simulink library "hdlsllibUNLOCKED"  (R2019a)
settings: Solver=ode45  StartTime=0.0  StopTime=10.0  RelTol=1e-3  EnableMultiTasking=on
values from neighbouring files (symbols this model uses):
  freerun = strcmp(get_param(blk, 'CountType'), 'Free running')    [hdlblkmask_counter.m]
  maxval_sc = countrange(2)    [hdlblkmask_counter.m]
  samptime = -1    [hdlblkmask_counter.m]
undefined symbols (not defined in the file or in its folder): a, b, c, Dialog, DiscIntNeverNeededParam, Floor, HDLStatusEnum, jsin, magnitude, message, Newton, NumBits1, NumBits2, Raphson, Slope1, Slope2
libraries: simulink x70, $bdroot x5, hdlmdlgenlib x1, hdlsllib_helper x1
(part 2 of 3)

== system hdlsllibUNLOCKED/Discrete/Unit Delay Enabled Resettable Synchronous ==
  u : Inport
  E : Inport  Port=2
  R : Inport  Port=3
  Unit Delay Enabled Resettable : Subsystem
  y : Outport
  wires:
  u/1 -> Unit Delay Enabled Resettable/1(u)
  E/1 -> Unit Delay Enabled Resettable/2(E)
  R/1 -> Unit Delay Enabled Resettable/3(R)
  Unit Delay Enabled Resettable/1(y) -> y/1

== system hdlsllibUNLOCKED/Discrete/Unit Delay Resettable Synchronous ==
  u : Inport
  R : Inport  Port=2
  Unit Delay Resettable : Subsystem
  y : Outport
  wires:
  u/1 -> Unit Delay Resettable/1(u)
  R/1 -> Unit Delay Resettable/2(R)
  Unit Delay Resettable/1(y) -> y/1

== system hdlsllibUNLOCKED/HDL Subsystems/Enabled Synchronous Subsystem ==
  In1 : Inport
  Enable : EnablePort
  State Control : StateControl  StateControl=Synchronous
  Out1 : Outport
  wires:
  In1/1 -> Out1/1

== system hdlsllibUNLOCKED/HDL Subsystems/Resettable Synchronous Subsystem ==
  In1 : Inport
  Reset : ResetPort  DisableCoverage=on  ResetTriggerType=level hold
  State Control : StateControl  StateControl=Synchronous
  Out1 : Outport
  wires:
  In1/1 -> Out1/1

== system hdlsllibUNLOCKED/HDL Subsystems/Synchronous Subsystem ==
  In1 : Inport
  State Control : StateControl  StateControl=Synchronous
  Out1 : Outport
  wires:
  In1/1 -> Out1/1

== system hdlsllibUNLOCKED/HDL Operations/Deserializer1D ==
  S : Inport
  Delay : Delay  DelayLength=1  InitialCondition=0
  EnumToIntConverter : MATLAB Function  TreatAsAtomicUnit=on
  HDL1DDs : MATLABSystem  System=hdl.deserializer1D  Ratio=Ratio  IdleCycles=IdleCycles  InitialCondition=0  StartInPortEnb=off  ValidInPortEnb=off  SimulateUsing=Code generation
      mask Type: hdl.deserializer1D
      mask Display:
      | disp(['Deserializer' char(10) '1D']);
      | port_label('input',1,'dataIn');
      | port_label('input',2,'startIn');
      | port_label('input',3,'validIn');
      | port_label('output',1,'dataOut');
      | port_label('output',2,'validOut');
  IntToEnumConverter : MATLAB Function  TreatAsAtomicUnit=on
  Terminator : Terminator
  const_startIn : Constant  OutDataTypeStr=boolean
  const_validIn : Constant  OutDataTypeStr=boolean
  rateTrans : RateTransition  OutPortSampleTimeOpt=Multiple of input port sample time  OutPortSampleTimeMultiple=1 + 0  OutPortSampleTime=1
  rateTrans1 : RateTransition  OutPortSampleTimeOpt=Multiple of input port sample time  OutPortSampleTimeMultiple=1 + 0  OutPortSampleTime=1
  P : Outport
  wires:
  Delay/1 -> IntToEnumConverter/1(dataIn)
  S/1 -> Delay/1, EnumToIntConverter/1(dataIn)
  rateTrans/1 -> P/1
  HDL1DDs/2 -> rateTrans1/1
  rateTrans1/1 -> Terminator/1
  EnumToIntConverter/1(deserializer_preProcessed) -> HDL1DDs/1
  HDL1DDs/1 -> IntToEnumConverter/2(dataOut)
  IntToEnumConverter/1(deserializer_PostProcessed) -> rateTrans/1
  const_startIn/1 -> HDL1DDs/2
  const_validIn/1 -> HDL1DDs/3

== system hdlsllibUNLOCKED/HDL Operations/Multiply-Accumulate ==
  a : Inport
  b : Inport  Port=2
  streamingMAC_with_counter : Subsystem  Commented=on  mask{initValueSetting=Dialog, initValue=initValue3, num_samples_internal=num_samples, typeinfo=Inherit: Inherit via back propagation, RndMeth=Floor}
      mask prompts: num_samples_internal "Number of Samples:"; typeinfo "Output data type:"; RndMeth "Integer rounding mode"
      mask init:
      | hdlblkmask_streaming_internal(gcb, initValueSetting, initValue, num_samples_internal)
      mask TypeOptions initValueSetting: Dialog | Input port
      mask Callback initValueSetting: hdlblkmask_streaming_internal_cb(gcb)
      mask TypeOptions RndMeth: Multiply-Add/RndMeth
      mask DialogControl Container3 Prompt: Data
      mask DialogControl Control2 Prompt: (Add text here)
      mask DialogControl Control3 Prompt: Source
      mask DialogControl Control4 Prompt: Value
      mask DialogControl Control5 Prompt: Bias:
  streamingMAC_without_counter : Subsystem  Commented=on  mask{initValueSetting=Dialog, initValue=initValue2, typeinfo=Inherit: Inherit via back propagation, RndMeth=Floor}
      mask prompts: typeinfo "Output data type:"; RndMeth "Integer rounding mode"
      mask init:
      | hdlblkmask_streaming_internal(gcb,initValueSetting,initValue)
      mask TypeOptions initValueSetting: Dialog | Input port
      mask Callback initValueSetting: hdlblkmask_streaming_internal_cb(gcb)
      mask TypeOptions RndMeth: Multiply-Add/RndMeth
      mask DialogControl Container3 Prompt: Data
      mask DialogControl Control2 Prompt: (Add text here)
      mask DialogControl Control3 Prompt: Source
      mask DialogControl Control4 Prompt: Value
      mask DialogControl Control5 Prompt: Bias:
  vectorMAC : Subsystem  mask{dim=-1, initValueSetting=Dialog, initValue=initValue, parallel=off, AccumDataTypeStr=Inherit: Inherit via internal rule, RndMeth=Floor, DoSatur=off}
      mask prompts: dim "Specify input dimensions"; parallel "Use fully parallel implementation"; AccumDataTypeStr "Simulink:blkprm_prompts:OUTPUT_UNIFIEDDATATYPE"; RndMeth "Simulink:blkprm_prompts:SPP_RndMeth_ID"; DoSatur "Simulink:blkprm_prompts:AllBlksSaturate"
      mask init:
      | hdlblkmask_mac(gcb, initValueSetting, initValue)
      mask TypeOptions initValueSetting: Dialog | Input port
      mask Callback initValueSetting: hdlblkmask_mac_cb(gcb);
      mask TypeOptions AccumDataTypeStr: Sum/AccumDataTypeStr
      mask TypeOptions RndMeth: Sum/RndMeth
      mask TypeOptions DoSatur: Sum/SaturateOnIntegerOverflow
      mask DialogControl Container3 Prompt: Data
      mask DialogControl Control3 Prompt: (Add text here)
      mask DialogControl Control4 Prompt: Source
      mask DialogControl Control5 Prompt: Value
      mask DialogControl Control2 Prompt: Bias:
      mask DialogControl AccumDataTypeStr Prompt: Output data type:
      mask DialogControl RndMeth Prompt: Integer rounding mode:
      mask DialogControl DoSatur Prompt: Saturate on integer overflow
      mask Display:
      | maskVal = get_param(gcb,'MaskValues');
      | initValueSetting = maskVal{2};
      | if(strcmp(initValueSetting,'Input port'))
      |     port_label('input', 1, 'a');
      |     port_label('input', 2, 'b');
      |     port_label('input', 3, 'c');
      |     disp([char(8721),'a(i)*b(i)+c'])
      | elseif(initValue ~= 0)
      |     port_label('input', 1, 'a');
      |     port_label('input', 2, 'b');
      |     disp([char(8721),'a(i)*b(i)+k'])
      | else
      |     port_label('input', 1, 'a');
      |     port_label('input', 2, 'b');
      |     disp([char(8721),'a(i)*b(i)'])
      | end
  dataOut : Outport
  wires:
  a/1 -> vectorMAC/1(In1)
  b/1 -> vectorMAC/2(In2)
  vectorMAC/1(Out1) -> dataOut/1

== system hdlsllibUNLOCKED/HDL Operations/Multiply-Add ==
  a : Inport
  b : Inport  Port=2
  c : Inport  Port=3
  Product : Product
  Sum : Sum  OutDataTypeStr=datatype
  Out : Outport
  wires:
  c/1 -> Sum/1
  a/1 -> Product/1
  b/1 -> Product/2
  Sum/1 -> Out/1
  Product/1 -> Sum/2

== system hdlsllibUNLOCKED/HDL Operations/Serializer1D ==
  P : Inport
  EnumToIntConverter : MATLAB Function  TreatAsAtomicUnit=on
  HDL1DSe : MATLABSystem  System=hdl.serializer1D  Ratio=Ratio  IdleCycles=IdleCycles  SimulateUsing=Code generation
      mask Type: hdl.serializer1D
      mask Display:
      | disp(['Serializer' char(10) '1D']);
      | port_label('input',1,'dataIn');
      | port_label('input',2,'validIn');
      | port_label('output',1,'dataOut');
      | port_label('output',2,'startOut');
      | port_label('output',3,'validOut');
  IntToEnumConverter : MATLAB Function  TreatAsAtomicUnit=on
  Terminator : Terminator
  Terminator1 : Terminator
  const_validIn : Constant  OutDataTypeStr=boolean
  rateTrans : RateTransition  Integrity=off  OutPortSampleTimeOpt=Multiple of input port sample time  OutPortSampleTimeMultiple=1/(1 + 0)  OutPortSampleTime=1
  rateTrans1 : RateTransition  Integrity=off  OutPortSampleTimeOpt=Multiple of input port sample time  OutPortSampleTimeMultiple=1/(1 + 0)  OutPortSampleTime=1
  S : Outport
  wires:
  P/1 -> rateTrans/1
  rateTrans/1 -> IntToEnumConverter/1(dataIn), EnumToIntConverter/1(dataIn)
  HDL1DSe/2 -> Terminator/1
  HDL1DSe/3 -> Terminator1/1
  rateTrans1/1 -> HDL1DSe/2
  const_validIn/1 -> rateTrans1/1
  EnumToIntConverter/1(serializer_preProcessed) -> HDL1DSe/1
  HDL1DSe/1 -> IntToEnumConverter/2(dataOut)
  IntToEnumConverter/1(serializer_PostProcessed) -> S/1

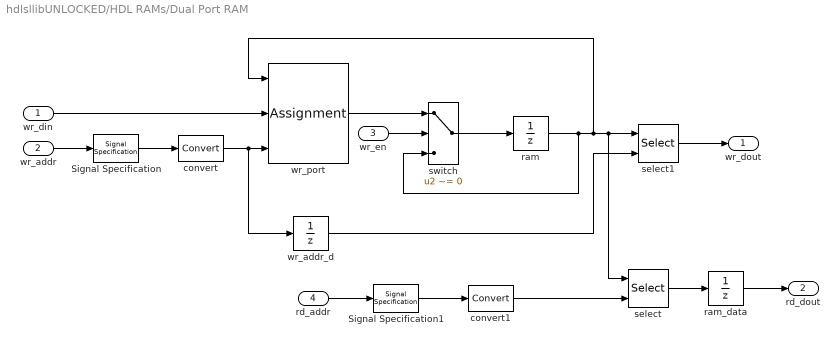
== system hdlsllibUNLOCKED/HDL RAMs/Dual Port RAM ==
  wr_din : Inport
  wr_addr : Inport  Port=2
  wr_en : Inport  Port=3  OutDataTypeStr=boolean
  rd_addr : Inport  Port=4
  Signal Specification : SignalSpecification  OutDataTypeStr=fixdt(0,ram_size,0)  Dimensions=1
  Signal Specification1 : SignalSpecification  OutDataTypeStr=fixdt(0,ram_size,0)  Dimensions=1
  convert : DataTypeConversion
  convert1 : DataTypeConversion
  ram : UnitDelay  SampleTime=-1  HasFrameUpgradeWarning=on
  ram_data : UnitDelay  SampleTime=-1  HasFrameUpgradeWarning=on
  select : Selector  IndexMode=Zero-based  InputPortWidth=2^ram_size  IndexOptions=Index vector (port)  Indices=[1 3]  OutputSizes=1
  select1 : Selector  IndexMode=Zero-based  InputPortWidth=2^ram_size  IndexOptions=Index vector (port)  Indices=[1 3]  OutputSizes=1
  switch : Switch  Criteria=u2 ~= 0
  wr_addr_d : UnitDelay  SampleTime=-1  HasFrameUpgradeWarning=on
  wr_port : Assignment  IndexMode=Zero-based  IndexOptions=Index vector (port)  Indices=1  OutputSizes=[1 1]
  wr_dout : Outport
  rd_dout : Outport  Port=2
  wires:
  Signal Specification1/1 -> convert1/1
  wr_addr_d/1 -> select1/2
  select1/1 -> wr_dout/1
  convert1/1 -> select/2
  convert/1 -> wr_addr_d/1, wr_port/3
  select/1 -> ram_data/1
  rd_addr/1 -> Signal Specification1/1
  wr_en/1 -> switch/2
  wr_din/1 -> wr_port/2
  ram/1 -> switch/3, select1/1, select/1, wr_port/1
  switch/1 -> ram/1
  wr_port/1 -> switch/1
  wr_addr/1 -> Signal Specification/1
  Signal Specification/1 -> convert/1
  ram_data/1 -> rd_dout/1

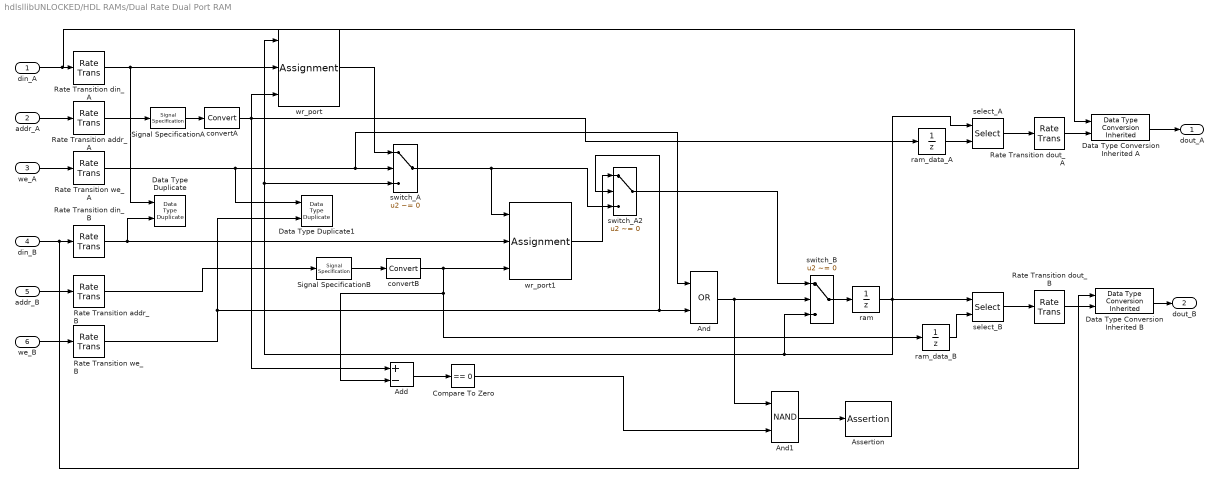
== system hdlsllibUNLOCKED/HDL RAMs/Dual Rate Dual Port RAM ==
  din_A : Inport
  addr_A : Inport  Port=2
  we_A : Inport  Port=3  OutDataTypeStr=boolean
  din_B : Inport  Port=4
  addr_B : Inport  Port=5
  we_B : Inport  Port=6  OutDataTypeStr=boolean
  Add : Sum  Inputs=+-
  And : Logic  Operator=OR  AllPortsSameDT=off  OutDataTypeStr=boolean
  And1 : Logic  Operator=NAND  AllPortsSameDT=off  OutDataTypeStr=boolean
  Assertion : Assertion
  Compare To Zero : simulink/Logic and Bit Operations/Compare To Zero  relop===  OutDataTypeStr=boolean
  Data Type Conversion Inherited A : simulink/Signal Attributes/Data Type Conversion Inherited  ConvertRealWorld=Real World Value  DoSatur=off
      settings: SourceProductName=Simulink  SourceProductBaseCode=SL
  Data Type Conversion Inherited B : simulink/Signal Attributes/Data Type Conversion Inherited  ConvertRealWorld=Real World Value  DoSatur=off
      settings: SourceProductName=Simulink  SourceProductBaseCode=SL
  Data Type Duplicate : DataTypeDuplicate
  Data Type Duplicate1 : DataTypeDuplicate
  Rate Transition addr_A : RateTransition  Integrity=off
  Rate Transition addr_B : RateTransition  Integrity=off
  Rate Transition din_A : RateTransition  Integrity=off
  Rate Transition din_B : RateTransition  Integrity=off
  Rate Transition dout_A : RateTransition  Integrity=off
  Rate Transition dout_B : RateTransition  Integrity=off
  Rate Transition we_A : RateTransition  Integrity=off
  Rate Transition we_B : RateTransition  Integrity=off
  Signal SpecificationA : SignalSpecification  OutDataTypeStr=fixdt(0,ram_size,0)  Dimensions=1
  Signal SpecificationB : SignalSpecification  OutDataTypeStr=fixdt(0,ram_size,0)  Dimensions=1
  convertA : DataTypeConversion
  convertB : DataTypeConversion
  ram : UnitDelay  SampleTime=-1  HasFrameUpgradeWarning=on
  ram_data_A : UnitDelay  SampleTime=-1  HasFrameUpgradeWarning=on
  ram_data_B : UnitDelay  SampleTime=-1  HasFrameUpgradeWarning=on
  select_A : Selector  IndexMode=Zero-based  InputPortWidth=2^ram_size  IndexOptions=Index vector (port)  Indices=[1 3]  OutputSizes=1
  select_B : Selector  IndexMode=Zero-based  InputPortWidth=2^ram_size  IndexOptions=Index vector (port)  Indices=[1 3]  OutputSizes=1
  switch_A : Switch  Criteria=u2 ~= 0
  switch_A2 : Switch  Criteria=u2 ~= 0
  switch_B : Switch  Criteria=u2 ~= 0
  wr_port : Assignment  IndexMode=Zero-based  IndexOptions=Index vector (port)  Indices=1  OutputSizes=[1 1]
  wr_port1 : Assignment  IndexMode=Zero-based  IndexOptions=Index vector (port)  Indices=1  OutputSizes=[1 1]
  dout_A : Outport
  dout_B : Outport  Port=2
  wires:
  we_A/1 -> Rate Transition we_A/1
  select_A/1 -> Rate Transition dout_A/1
  switch_A2/1 -> switch_B/1
  And1/1 -> Assertion/1
  Signal SpecificationA/1 -> convertA/1
  Signal SpecificationB/1 -> convertB/1
  din_B/1 -> Data Type Conversion Inherited B/1, Rate Transition din_B/1
  switch_B/1 -> ram/1
  addr_B/1 -> Rate Transition addr_B/1
  convertA/1 -> ram_data_A/1, wr_port/3, Add/1
  we_B/1 -> Rate Transition we_B/1
  ram/1 -> select_B/1, switch_B/3, switch_A/3, wr_port/1, select_A/1
  wr_port/1 -> switch_A/1
  And/1 -> And1/1, switch_B/2
  wr_port1/1 -> switch_A2/1
  Add/1 -> Compare To Zero/1
  Compare To Zero/1 -> And1/2
  Rate Transition we_B/1 -> switch_A2/2, And/2, Data Type Duplicate1/2
  switch_A/1 -> wr_port1/1, switch_A2/3
  Rate Transition addr_B/1 -> Signal SpecificationB/1
  select_B/1 -> Rate Transition dout_B/1
  ram_data_B/1 -> select_B/2
  Rate Transition we_A/1 -> Data Type Duplicate1/1, And/1, switch_A/2
  ram_data_A/1 -> select_A/2
  Rate Transition din_A/1 -> Data Type Duplicate/1, wr_port/2
  convertB/1 -> ram_data_B/1, Add/2, wr_port1/3
  din_A/1 -> Data Type Conversion Inherited A/1, Rate Transition din_A/1
  Rate Transition din_B/1 -> wr_port1/2, Data Type Duplicate/2
  addr_A/1 -> Rate Transition addr_A/1
  Rate Transition addr_A/1 -> Signal SpecificationA/1
  Rate Transition dout_B/1 -> Data Type Conversion Inherited B/2
  Data Type Conversion Inherited B/1 -> dout_B/1
  Rate Transition dout_A/1 -> Data Type Conversion Inherited A/2
  Data Type Conversion Inherited A/1 -> dout_A/1

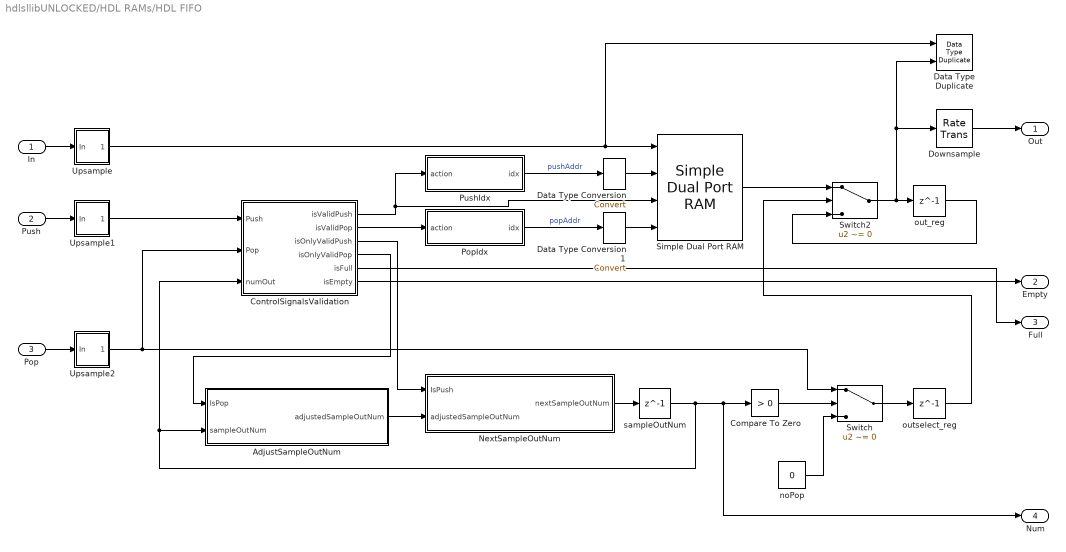
== system hdlsllibUNLOCKED/HDL RAMs/HDL FIFO ==
  In : Inport  PortDimensions=1
  Push : Inport  Port=2  PortDimensions=1
  Pop : Inport  Port=3  PortDimensions=1
  AdjustSampleOutNum : Subsystem
  Compare To Zero : simulink/Logic and Bit Operations/Compare To Zero  relop=>  OutDataTypeStr=boolean
  ControlSignalsValidation : Subsystem
  Data Type Duplicate : DataTypeDuplicate
  Data Type Conversion : DataTypeConversion
  Data Type Conversion1 : DataTypeConversion
  Downsample : RateTransition  OutPortSampleTimeOpt=Multiple of input port sample time  OutPortSampleTimeMultiple=ratio
  NextSampleOutNum : Subsystem
  PopIdx : Subsystem
  PushIdx : Subsystem
  Simple Dual Port RAM : $bdroot/HDL RAMs/Simple Dual Port RAM  ram_size=4
  Switch : Switch  Criteria=u2 ~= 0
  Switch2 : Switch  Criteria=u2 ~= 0
  Upsample : Subsystem
  Upsample1 : Subsystem
  Upsample2 : Subsystem
  noPop : Constant  Value=0
  out_reg : Delay  DelayLength=1  InitialCondition=0
  outselect_reg : Delay  DelayLength=1  InitialCondition=0
  sampleOutNum : Delay  DelayLength=1  InitialCondition=0
  Out : Outport  PortDimensions=1
  Empty : Outport  Port=2  PortDimensions=1
  Full : Outport  Port=3  PortDimensions=1
  Num : Outport  Port=4  PortDimensions=1
  wires:
  Downsample/1 -> Out/1
  Upsample2/1(Out) -> ControlSignalsValidation/2(Pop), Switch/1
  Upsample1/1(Out) -> ControlSignalsValidation/1(Push)
  Upsample/1(Out) -> Data Type Duplicate/1, Simple Dual Port RAM/1
  Simple Dual Port RAM/1 -> Switch2/1
  sampleOutNum/1 -> ControlSignalsValidation/3(numOut), AdjustSampleOutNum/2(sampleOutNum), Num/1, Compare To Zero/1
  AdjustSampleOutNum/1(adjustedSampleOutNum) -> NextSampleOutNum/2(adjustedSampleOutNum)
  NextSampleOutNum/1(nextSampleOutNum) -> sampleOutNum/1
  ControlSignalsValidation/2(isValidPop) -> PopIdx/1(action)
  out_reg/1 -> Switch2/3
  In/1 -> Upsample/1(In)
  outselect_reg/1 -> Switch2/2
  Switch/1 -> outselect_reg/1
  PushIdx/1(idx) -> Data Type Conversion/1  "pushAddr"
  PopIdx/1(idx) -> Data Type Conversion1/1  "popAddr"
  Switch2/1 -> Data Type Duplicate/2, Downsample/1, out_reg/1
  Compare To Zero/1 -> Switch/2
  noPop/1 -> Switch/3
  ControlSignalsValidation/4(isOnlyValidPop) -> AdjustSampleOutNum/1(IsPop)
  ControlSignalsValidation/5(isFull) -> Full/1
  ControlSignalsValidation/3(isOnlyValidPush) -> NextSampleOutNum/1(IsPush)
  ControlSignalsValidation/6(isEmpty) -> Empty/1
  Data Type Conversion1/1 -> Simple Dual Port RAM/4
  Data Type Conversion/1 -> Simple Dual Port RAM/2
  ControlSignalsValidation/1(isValidPush) -> PushIdx/1(action), Simple Dual Port RAM/3
  Push/1 -> Upsample1/1(In)
  Pop/1 -> Upsample2/1(In)

== system hdlsllibUNLOCKED/HDL RAMs/Simple Dual Port RAM ==
  wr_din : Inport
  wr_addr : Inport  Port=2
  wr_en : Inport  Port=3  OutDataTypeStr=boolean
  rd_addr : Inport  Port=4
  Signal Specification : SignalSpecification  OutDataTypeStr=fixdt(0,ram_size,0)  Dimensions=1
  Signal Specification1 : SignalSpecification  OutDataTypeStr=fixdt(0,ram_size,0)  Dimensions=1
  convert : DataTypeConversion
  convert1 : DataTypeConversion
  ram : UnitDelay  SampleTime=-1  HasFrameUpgradeWarning=on
  ram_data : UnitDelay  SampleTime=-1  HasFrameUpgradeWarning=on
  select : Selector  IndexMode=Zero-based  InputPortWidth=2^ram_size  IndexOptions=Index vector (port)  Indices=[1 3]  OutputSizes=1
  switch : Switch  Criteria=u2 ~= 0
  wr_port : Assignment  IndexMode=Zero-based  IndexOptions=Index vector (port)  Indices=1  OutputSizes=[1 1]
  rd_dout : Outport
  wires:
  wr_port/1 -> switch/1
  switch/1 -> ram/1
  ram/1 -> wr_port/1, select/1, switch/3
  wr_din/1 -> wr_port/2
  wr_en/1 -> switch/2
  wr_addr/1 -> Signal Specification/1
  rd_addr/1 -> Signal Specification1/1
  select/1 -> ram_data/1
  convert/1 -> wr_port/3
  convert1/1 -> select/2
  Signal Specification/1 -> convert/1
  Signal Specification1/1 -> convert1/1
  ram_data/1 -> rd_dout/1

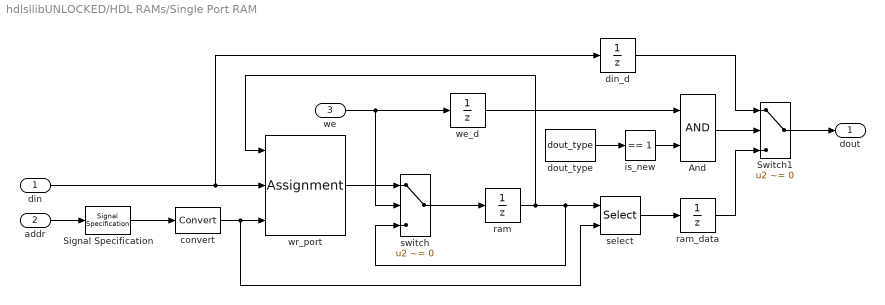
== system hdlsllibUNLOCKED/HDL RAMs/Single Port RAM ==
  din : Inport
  addr : Inport  Port=2
  we : Inport  Port=3  OutDataTypeStr=boolean
  And : Logic  AllPortsSameDT=off  OutDataTypeStr=boolean
  Signal Specification : SignalSpecification  OutDataTypeStr=fixdt(0,ram_size,0)  Dimensions=1
  Switch1 : Switch  Criteria=u2 ~= 0
  convert : DataTypeConversion
  din_d : UnitDelay  SampleTime=-1  HasFrameUpgradeWarning=on
  dout_type : Constant  Value=dout_type
  is_new : simulink/Logic and Bit Operations/Compare To Constant  relop===  const=1  OutDataTypeStr=boolean  ZeroCross=off
  ram : UnitDelay  SampleTime=-1  HasFrameUpgradeWarning=on
  ram_data : UnitDelay  SampleTime=-1  HasFrameUpgradeWarning=on
  select : Selector  IndexMode=Zero-based  InputPortWidth=2^ram_size  IndexOptions=Index vector (port)  Indices=[1 3]  OutputSizes=1
  switch : Switch  Criteria=u2 ~= 0
  we_d : UnitDelay  SampleTime=-1  HasFrameUpgradeWarning=on
  wr_port : Assignment  IndexMode=Zero-based  IndexOptions=Index vector (port)  Indices=1  OutputSizes=[1 1]
  dout : Outport
  wires:
  wr_port/1 -> switch/1
  switch/1 -> ram/1
  ram/1 -> switch/3, wr_port/1, select/1
  din/1 -> wr_port/2, din_d/1
  we/1 -> switch/2, we_d/1
  addr/1 -> Signal Specification/1
  select/1 -> ram_data/1
  convert/1 -> wr_port/3, select/2
  Signal Specification/1 -> convert/1
  Switch1/1 -> dout/1
  din_d/1 -> Switch1/1
  And/1 -> Switch1/2
  ram_data/1 -> Switch1/3
  dout_type/1 -> is_new/1
  is_new/1 -> And/2
  we_d/1 -> And/1

== system hdlsllibUNLOCKED/Logic and Bit Operations/Bit Concat ==
  u1 : Inport
  u2 : Inport  Port=2
  Bit Concat2 : hdlmdlgenlib/Bit Concat2
      settings: SourceProductName=Simulink  SourceProductBaseCode=SL
  y : Outport
  wires:
  Bit Concat2/1 -> y/1
  u1/1 -> Bit Concat2/1
  u2/1 -> Bit Concat2/2

== system hdlsllibUNLOCKED/Logic and Bit Operations/Bit Reduce ==
  u : Inport
  bit_reduce : MATLAB Function
  y : Outport
  wires:
  bit_reduce/1(y) -> y/1
  u/1 -> bit_reduce/1(u)

== system hdlsllibUNLOCKED/Logic and Bit Operations/Bit Rotate ==
  u : Inport
  bit_rotate : MATLAB Function
  y : Outport
  wires:
  bit_rotate/1(y) -> y/1
  u/1 -> bit_rotate/1(u)

== system hdlsllibUNLOCKED/Logic and Bit Operations/Bit Shift ==
  u : Inport
  bit_shift : MATLAB Function
  y : Outport
  wires:
  u/1 -> bit_shift/1(u)
  bit_shift/1(y) -> y/1

== system hdlsllibUNLOCKED/Logic and Bit Operations/Bit Slice ==
  u : Inport
  bit_slice : MATLAB Function
  y : Outport
  wires:
  u/1 -> bit_slice/1(u)
  bit_slice/1(y) -> y/1

== system hdlsllibUNLOCKED/Lookup Tables/Cosine HDL Optimized ==
  u : Inport
  cosine hdl : hdlsllib_helper/Cosine HDL Optimized  NumDataPoints=64  TableDataTypeStr=fixdt(0,16,15)  SimulateLUTROMDelay=off
      settings: SourceProductName=Simulink  SourceProductBaseCode=SL
  x : Outport
  wires:
  u/1 -> cosine hdl/1
  cosine hdl/1 -> x/1

== system hdlsllibUNLOCKED/Ports & Subsystems/Enabled Subsystem ==
  In1 : Inport
  Enable : EnablePort
  Out1 : Outport  InitialOutput=0
  wires:
  In1/1 -> Out1/1

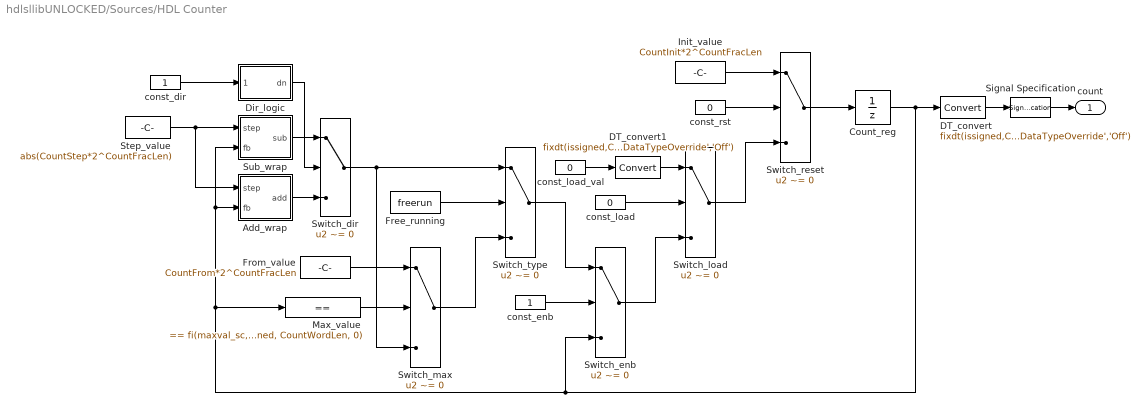
== system hdlsllibUNLOCKED/Sources/HDL Counter ==
  Add_wrap : Subsystem
  Count_reg : UnitDelay  InitialCondition=CountInit*2^CountFracLen  SampleTime=samptime  HasFrameUpgradeWarning=on
  DT_convert : DataTypeConversion  OutDataTypeStr=fixdt(issigned,CountWordLen,CountFracLen,'DataTypeOverride','Off')  ConvertRealWorld=Stored Integer (SI)
  DT_convert1 : DataTypeConversion  OutDataTypeStr=fixdt(issigned,CountWordLen,0,'DataTypeOverride','Off')  ConvertRealWorld=Stored Integer (SI)
  Dir_logic : Subsystem
  Free_running : Constant  Value=freerun  OutDataTypeStr=boolean
  From_value : Constant  Value=CountFrom*2^CountFracLen  OutDataTypeStr=fixdt(issigned,CountWordLen, 0,'DataTypeOverride','Off')
  Init_value : Constant  Value=CountInit*2^CountFracLen  OutDataTypeStr=fixdt(issigned,CountWordLen, 0,'DataTypeOverride','Off')
  Max_value : simulink/Logic and Bit Operations/Compare To Constant  relop===  const=fi(maxval_sc, issigned, CountWordLen, 0)  OutDataTypeStr=boolean  ZeroCross=off
  Signal Specification : SignalSpecification  Dimensions=1
  Step_value : Constant  Value=abs(CountStep*2^CountFracLen)  OutDataTypeStr=fixdt(issigned,CountWordLen,0,'DataTypeOverride','Off')
  Sub_wrap : Subsystem
  Switch_dir : Switch  Criteria=u2 ~= 0
  Switch_enb : Switch  Criteria=u2 ~= 0
  Switch_load : Switch  Criteria=u2 ~= 0
  Switch_max : Switch  Criteria=u2 ~= 0
  Switch_reset : Switch  Criteria=u2 ~= 0  OutDataTypeStr=fixdt(issigned,CountWordLen, 0,'DataTypeOverride','Off')
  Switch_type : Switch  Criteria=u2 ~= 0
  const_dir : Constant  OutDataTypeStr=boolean
  const_enb : Constant  OutDataTypeStr=boolean
  const_load : Constant  Value=0  OutDataTypeStr=boolean
  const_load_val : Constant  Value=0  OutDataTypeStr=fixdt(issigned,CountWordLen,CountFracLen,'DataTypeOverride','Off')
  const_rst : Constant  Value=0  OutDataTypeStr=boolean
  count : Outport
  wires:
  Signal Specification/1 -> count/1
  DT_convert1/1 -> Switch_load/1
  Dir_logic/1(dn) -> Switch_dir/2
  Sub_wrap/1(sub) -> Switch_dir/1
  Add_wrap/1(add) -> Switch_dir/3
  DT_convert/1 -> Signal Specification/1
  Free_running/1 -> Switch_type/2
  Switch_max/1 -> Switch_type/3
  From_value/1 -> Switch_max/1
  Max_value/1 -> Switch_max/2
  Switch_type/1 -> Switch_enb/1
  Step_value/1 -> Sub_wrap/1(step), Add_wrap/1(step)
  const_dir/1 -> Dir_logic/1(dir_port)
  const_enb/1 -> Switch_enb/2
  Switch_enb/1 -> Switch_load/3
  const_load_val/1 -> DT_convert1/1
  const_load/1 -> Switch_load/2
  Switch_load/1 -> Switch_reset/3
  Count_reg/1 -> DT_convert/1, Add_wrap/2(fb), Sub_wrap/2(fb), Max_value/1, Switch_enb/3
  Switch_reset/1 -> Count_reg/1
  const_rst/1 -> Switch_reset/2
  Init_value/1 -> Switch_reset/1
  Switch_dir/1 -> Switch_max/3, Switch_type/1

== system hdlsllibUNLOCKED/Discrete/Unit Delay Enabled Synchronous/Unit Delay Enabled ==
  u : Inport
  E : Inport  Port=2
  Enabled Delay : Delay  DelayLength=1  InitialCondition=InitialCondition  ShowEnablePort=on  SampleTime=SampleTime
      settings: InputPortMap=u0,e6
  State Control : StateControl  StateControl=Synchronous
  y : Outport
  wires:
  Enabled Delay/1 -> y/1
  u/1 -> Enabled Delay/1
  E/1 -> Enabled Delay/2

== system hdlsllibUNLOCKED/Discrete/Unit Delay Enabled Resettable Synchronous/Unit Delay Enabled Resettable ==
  u : Inport
  E : Inport  Port=2
  R : Inport  Port=3
  Enabled Resettable Delay : Delay  DelayLength=1  InitialCondition=InitialCondition  ExternalReset=Level hold  ShowEnablePort=on  SampleTime=SampleTime
      settings: InputPortMap=u0,e6,r5
  State Control : StateControl  StateControl=Synchronous
  y : Outport
  wires:
  Enabled Resettable Delay/1 -> y/1
  E/1 -> Enabled Resettable Delay/2
  u/1 -> Enabled Resettable Delay/1
  R/1 -> Enabled Resettable Delay/3

== system hdlsllibUNLOCKED/Discrete/Unit Delay Resettable Synchronous/Unit Delay Resettable ==
  u : Inport
  R : Inport  Port=2
  Resettable Delay : Delay  DelayLength=1  InitialCondition=InitialCondition  ExternalReset=Level hold  SampleTime=SampleTime
      settings: InputPortMap=u0,r5
  State Control : StateControl  StateControl=Synchronous
  y : Outport
  wires:
  u/1 -> Resettable Delay/1
  R/1 -> Resettable Delay/2
  Resettable Delay/1 -> y/1

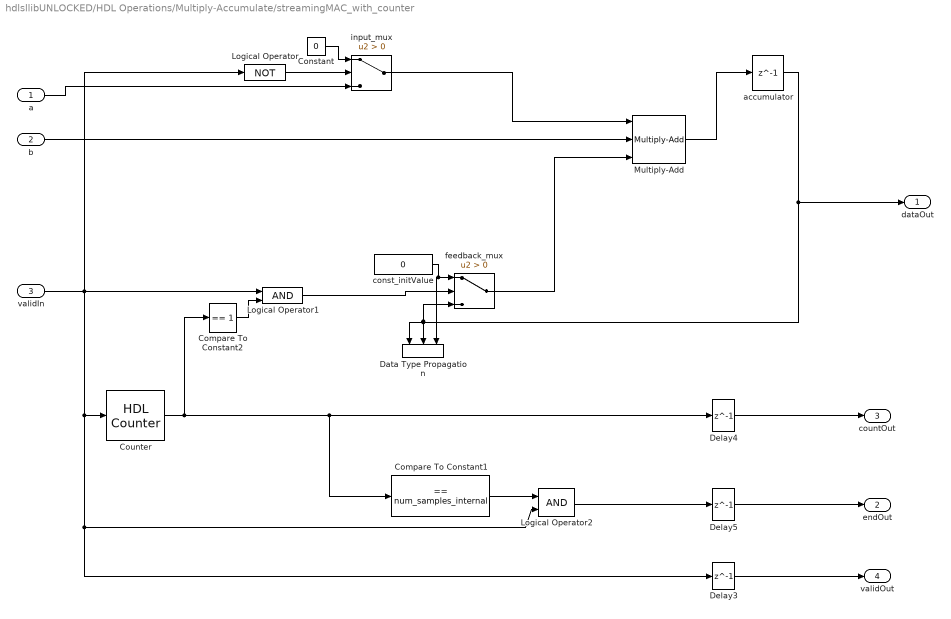
== system hdlsllibUNLOCKED/HDL Operations/Multiply-Accumulate/streamingMAC_with_counter ==
  "a " : Inport
  "b " : Inport  Port=2
  validIn : Inport  Port=3
  Compare To Constant1 : simulink/Logic and Bit Operations/Compare To Constant  relop===  const=num_samples_internal  OutDataTypeStr=boolean
  Compare To Constant2 : simulink/Logic and Bit Operations/Compare To Constant  relop===  const=1  OutDataTypeStr=boolean
  Constant : Constant  Value=0  OutDataTypeStr=Inherit: Inherit via back propagation  SampleTime=-1
  Counter : $bdroot/Sources/HDL Counter  CountType=Count limited  CountInit=1  CountStep=1  CountMax=num_samples_internal  CountFromType=Initial value  CountFrom=1  CountResetPort=off  CountLoadPort=off  CountEnbPort=on  CountDirPort=off  CountDataType=Unsigned  CountWordLen=2  CountFracLen=0  CountSampTime=1
  Data Type Propagation : simulink/Signal Attributes/Data Type Propagation  PropDataType=fixdt(1, 16)  IfRefDouble=double  IfRefSingle=single  IsSigned=IsSigned1 or IsSigned2  NumBitsBase=max([NumBits1 NumBits2])  NumBitsMult=1  NumBitsAdd=0  NumBitsAllowFinal=1:128  PropScaling=2^-10  ValuesUsedBestPrec=[5 -7]  SlopeBase=min([Slope1 Slope2])  SlopeMult=1  SlopeAdd=0  BiasBase=Bias1  BiasMult=1  BiasAdd=0
      settings: SourceProductName=Simulink  SourceProductBaseCode=SL
  Delay3 : Delay  DelayLength=1  InitialCondition=0
  Delay4 : Delay  DelayLength=1  InitialCondition=1
  Delay5 : Delay  DelayLength=1  InitialCondition=0
  Logical Operator : Logic  Operator=NOT  AllPortsSameDT=off  OutDataTypeStr=boolean
  Logical Operator1 : Logic  AllPortsSameDT=off  OutDataTypeStr=boolean
  Logical Operator2 : Logic  AllPortsSameDT=off  OutDataTypeStr=boolean
  Multiply-Add : $bdroot/HDL Operations/Multiply-Add  Function=c+(a.*b)  datatype=typeinfo  DoSatur=off  FMA=off
  accumulator : Delay  DelayLength=1  InitialCondition=0
  const_initValue : Constant  Value=0  OutDataTypeStr=Inherit: Inherit via back propagation  SampleTime=-1
  feedback_mux : Switch  Criteria=u2 > Threshold
  input_mux : Switch  Criteria=u2 > Threshold
  dataOut : Outport
  endOut : Outport  Port=2
  countOut : Outport  Port=3
  validOut : Outport  Port=4
  wires:
  Compare To Constant2/1 -> Logical Operator1/2
  Counter/1 -> Compare To Constant2/1, Compare To Constant1/1, Delay4/1
  validIn/1 -> Logical Operator2/2, Delay3/1, Counter/1, Logical Operator1/1, Logical Operator/1
  input_mux/1 -> Multiply-Add/1
  Delay4/1 -> countOut/1
  Compare To Constant1/1 -> Logical Operator2/1
  Constant/1 -> input_mux/1
  Delay5/1 -> endOut/1
  const_initValue/1 -> Data Type Propagation/3, feedback_mux/1
  feedback_mux/1 -> Multiply-Add/3
  Delay3/1 -> validOut/1
  Multiply-Add/1 -> accumulator/1
  Logical Operator1/1 -> feedback_mux/2
  Logical Operator/1 -> input_mux/2
  "a "/1 -> input_mux/3
  "b "/1 -> Multiply-Add/2
  Logical Operator2/1 -> Delay5/1
  accumulator/1 -> dataOut/1, Data Type Propagation/1, Data Type Propagation/2, feedback_mux/3

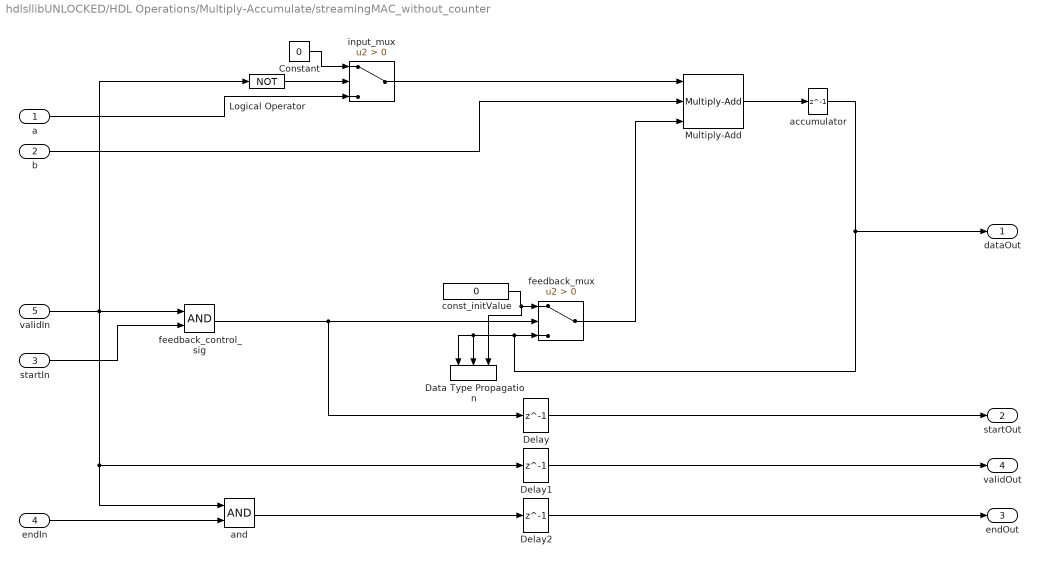
== system hdlsllibUNLOCKED/HDL Operations/Multiply-Accumulate/streamingMAC_without_counter ==
  "a " : Inport
  "b " : Inport  Port=2
  startIn : Inport  Port=3
  endIn : Inport  Port=4
  validIn : Inport  Port=5
  Constant : Constant  Value=0  OutDataTypeStr=Inherit: Inherit via back propagation  SampleTime=-1
  Data Type Propagation : simulink/Signal Attributes/Data Type Propagation  PropDataType=fixdt(1, 16)  IfRefDouble=double  IfRefSingle=single  IsSigned=IsSigned1 or IsSigned2  NumBitsBase=max([NumBits1 NumBits2])  NumBitsMult=1  NumBitsAdd=0  NumBitsAllowFinal=1:128  PropScaling=2^-10  ValuesUsedBestPrec=[5 -7]  SlopeBase=min([Slope1 Slope2])  SlopeMult=1  SlopeAdd=0  BiasBase=Bias1  BiasMult=1  BiasAdd=0
      settings: SourceProductName=Simulink  SourceProductBaseCode=SL
  Delay : Delay  DelayLength=1
  Delay1 : Delay  DelayLength=1
  Delay2 : Delay  DelayLength=1
  Logical Operator : Logic  Operator=NOT  AllPortsSameDT=off  OutDataTypeStr=boolean
  Multiply-Add : $bdroot/HDL Operations/Multiply-Add  Function=c+(a.*b)  datatype=typeinfo  DoSatur=off  FMA=off
  accumulator : Delay  DelayLength=1  InitialCondition=0
  and : Logic  AllPortsSameDT=off  OutDataTypeStr=boolean
  const_initValue : Constant  Value=0  OutDataTypeStr=Inherit: Inherit via back propagation  SampleTime=-1
  feedback_control_sig : Logic  AllPortsSameDT=off  OutDataTypeStr=boolean
  feedback_mux : Switch  Criteria=u2 > Threshold
  input_mux : Switch  Criteria=u2 > Threshold
  dataOut : Outport
  startOut : Outport  Port=2
  endOut : Outport  Port=3
  validOut : Outport  Port=4
  wires:
  "b "/1 -> Multiply-Add/2
  Multiply-Add/1 -> accumulator/1
  startIn/1 -> feedback_control_sig/2
  Constant/1 -> input_mux/1
  Logical Operator/1 -> input_mux/2
  input_mux/1 -> Multiply-Add/1
  "a "/1 -> input_mux/3
  feedback_mux/1 -> Multiply-Add/3
  feedback_control_sig/1 -> Delay/1, feedback_mux/2
  const_initValue/1 -> Data Type Propagation/3, feedback_mux/1
  validIn/1 -> and/1, Delay1/1, feedback_control_sig/1, Logical Operator/1
  Delay/1 -> startOut/1
  Delay1/1 -> validOut/1
  Delay2/1 -> endOut/1
  and/1 -> Delay2/1
  endIn/1 -> and/2
  accumulator/1 -> dataOut/1, feedback_mux/3, Data Type Propagation/2, Data Type Propagation/1

== system hdlsllibUNLOCKED/HDL Operations/Multiply-Accumulate/vectorMAC ==
  In1 : Inport
  In2 : Inport  Port=2
  Add : Subsystem  VariantControlMode=Label  Variant=on  LabelModeActiveChoice=zeroInitVal
  Constant : Constant  Value=0  OutDataTypeStr=Inherit: Inherit via back propagation  SampleTime=-1
  Data Type Propagation : simulink/Signal Attributes/Data Type Propagation  PropDataType=fixdt(1, 16)  IfRefDouble=double  IfRefSingle=single  IsSigned=IsSigned1 or IsSigned2  NumBitsBase=max([NumBits1 NumBits2])  NumBitsMult=1  NumBitsAdd=0  NumBitsAllowFinal=1:128  PropScaling=2^-10  ValuesUsedBestPrec=[5 -7]  SlopeBase=min([Slope1 Slope2])  SlopeMult=1  SlopeAdd=0  BiasBase=Bias1  BiasMult=1  BiasAdd=0
      settings: SourceProductName=Simulink  SourceProductBaseCode=SL
  Product : Product
  Reshape : Reshape
  Reshape1 : Reshape
  Reshape2 : Reshape
  Sum : Sum  Inputs=+  OutDataTypeStr=Inherit: Same as accumulator
  Out1 : Outport
  wires:
  Reshape1/1 -> Product/2
  Reshape2/1 -> Add/2(In2), Data Type Propagation/3
  Add/1(Out1) -> Out1/1
  Sum/1 -> Add/1(In1), Data Type Propagation/1, Data Type Propagation/2
  Product/1 -> Sum/1
  Reshape/1 -> Product/1
  In1/1 -> Reshape/1
  Constant/1 -> Reshape2/1
  In2/1 -> Reshape1/1

== system hdlsllibUNLOCKED/HDL RAMs/HDL FIFO/AdjustSampleOutNum ==
  IsPop : Inport
  sampleOutNum : Inport  Port=2
  AddSatOff : Subsystem  mask(Add){OutDataTypeStr=fixdt(0,4,0,'DataTypeOverride', 'Off')}
      mask prompts: OutDataTypeStr "Output data type :"
      mask help: Add inputs. Overflows wrap to the minimum value that is representableby the data type.
      mask init:
      | hdlblkmask_fifo('addwrapoverflow');
      mask Display:
      | portsInfo = get_param(gcb, 'ports');
      | numIn = portsInfo(1);
      | for ii=1:numIn
      |     port_label('input',ii,'+')
      | end
  NumConstant : Constant  Value=15  OutDataTypeStr=fixdt(0,4,0,'DataTypeOverride', 'Off')
  Switch : Switch  Criteria=u2 ~= 0
  adjustedSampleOutNum : Outport
  wires:
  NumConstant/1 -> AddSatOff/1(In1)
  AddSatOff/1(Out) -> Switch/1
  IsPop/1 -> Switch/2
  sampleOutNum/1 -> Switch/3, AddSatOff/2(In2)
  Switch/1 -> adjustedSampleOutNum/1

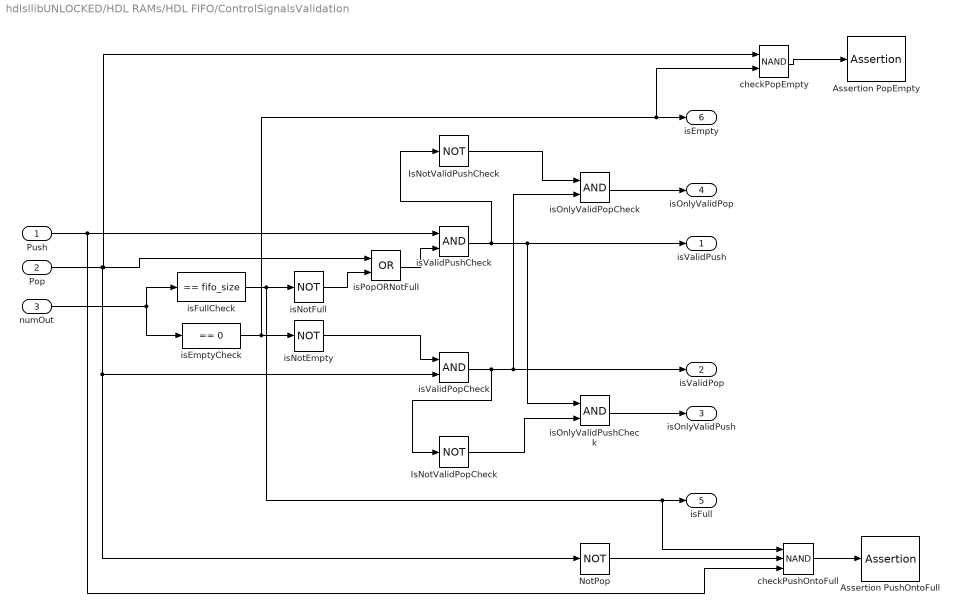
== system hdlsllibUNLOCKED/HDL RAMs/HDL FIFO/ControlSignalsValidation ==
  Push : Inport
  Pop : Inport  Port=2
  numOut : Inport  Port=3
  Assertion PopEmpty : Assertion  AssertionFailFcn=warning(message('hdlsllib:hdlsllib:FIFOPopEmpty'))  StopWhenAssertionFail=off
  Assertion PushOntoFull : Assertion  AssertionFailFcn=warning(message('hdlsllib:hdlsllib:FIFOPushFull'))  StopWhenAssertionFail=off
  IsNotValidPopCheck : Logic  Operator=NOT  AllPortsSameDT=off  OutDataTypeStr=boolean
  IsNotValidPushCheck : Logic  Operator=NOT  AllPortsSameDT=off  OutDataTypeStr=boolean
  NotPop : Logic  Operator=NOT  AllPortsSameDT=off  OutDataTypeStr=boolean
  checkPopEmpty : Logic  Operator=NAND  AllPortsSameDT=off  OutDataTypeStr=boolean
  checkPushOntoFull : Logic  Operator=NAND  Inputs=3  AllPortsSameDT=off  OutDataTypeStr=boolean
  isEmptyCheck : simulink/Logic and Bit Operations/Compare To Zero  relop===  OutDataTypeStr=boolean
  isFullCheck : simulink/Logic and Bit Operations/Compare To Constant  relop===  const=fifo_size  OutDataTypeStr=boolean
  isNotEmpty : Logic  Operator=NOT  AllPortsSameDT=off  OutDataTypeStr=boolean
  isNotFull : Logic  Operator=NOT  AllPortsSameDT=off  OutDataTypeStr=boolean
  isOnlyValidPopCheck : Logic  AllPortsSameDT=off  OutDataTypeStr=boolean
  isOnlyValidPushCheck : Logic  AllPortsSameDT=off  OutDataTypeStr=boolean
  isPopORNotFull : Logic  Operator=OR  AllPortsSameDT=off  OutDataTypeStr=boolean
  isValidPopCheck : Logic  AllPortsSameDT=off  OutDataTypeStr=boolean
  isValidPushCheck : Logic  AllPortsSameDT=off  OutDataTypeStr=boolean
  isValidPush : Outport
  isValidPop : Outport  Port=2
  isOnlyValidPush : Outport  Port=3
  isOnlyValidPop : Outport  Port=4
  isFull : Outport  Port=5
  isEmpty : Outport  Port=6
  wires:
  isEmptyCheck/1 -> isEmpty/1, checkPopEmpty/2, isNotEmpty/1
  checkPopEmpty/1 -> Assertion PopEmpty/1
  checkPushOntoFull/1 -> Assertion PushOntoFull/1
  IsNotValidPopCheck/1 -> isOnlyValidPushCheck/2
  Push/1 -> isValidPushCheck/1, checkPushOntoFull/3
  numOut/1 -> isEmptyCheck/1, isFullCheck/1
  isPopORNotFull/1 -> isValidPushCheck/2
  isFullCheck/1 -> checkPushOntoFull/1, isFull/1, isNotFull/1
  isNotFull/1 -> isPopORNotFull/2
  isValidPushCheck/1 -> isValidPush/1, isOnlyValidPushCheck/1, IsNotValidPushCheck/1
  isNotEmpty/1 -> isValidPopCheck/1
  isValidPopCheck/1 -> isOnlyValidPopCheck/2, isValidPop/1, IsNotValidPopCheck/1
  Pop/1 -> NotPop/1, isValidPopCheck/2, isPopORNotFull/1, checkPopEmpty/1
  isOnlyValidPushCheck/1 -> isOnlyValidPush/1
  IsNotValidPushCheck/1 -> isOnlyValidPopCheck/1
  isOnlyValidPopCheck/1 -> isOnlyValidPop/1
  NotPop/1 -> checkPushOntoFull/2

== system hdlsllibUNLOCKED/HDL RAMs/HDL FIFO/NextSampleOutNum ==
  IsPush : Inport
  adjustedSampleOutNum : Inport  Port=2
  AddSatOff : Subsystem  mask(Add){OutDataTypeStr=fixdt(0,4,0,'DataTypeOverride', 'Off')}
      mask prompts: OutDataTypeStr "Output data type :"
      mask help: Add inputs. Overflows wrap to the minimum value that is representableby the data type.
      mask init:
      | hdlblkmask_fifo('addwrapoverflow');
      mask Display:
      | portsInfo = get_param(gcb, 'ports');
      | numIn = portsInfo(1);
      | for ii=1:numIn
      |     port_label('input',ii,'+')
      | end
  IncrConstant : Constant  OutDataTypeStr=fixdt(0,4,0,'DataTypeOverride', 'Off')
  Switch : Switch  Criteria=u2 ~= 0
  nextSampleOutNum : Outport
  wires:
  Switch/1 -> nextSampleOutNum/1
  adjustedSampleOutNum/1 -> Switch/3, AddSatOff/2(In2)
  IsPush/1 -> Switch/2
  AddSatOff/1(Out) -> Switch/1
  IncrConstant/1 -> AddSatOff/1(In1)

== system hdlsllibUNLOCKED/HDL RAMs/HDL FIFO/PopIdx ==
  action : Inport
  AddSatOff : Subsystem  mask(Add){OutDataTypeStr=fixdt(0,4,0,'DataTypeOverride', 'Off')}
      mask prompts: OutDataTypeStr "Output data type :"
      mask help: Add inputs. Overflows wrap to the minimum value that is representableby the data type.
      mask init:
      | hdlblkmask_fifo('addwrapoverflow');
      mask Display:
      | portsInfo = get_param(gcb, 'ports');
      | numIn = portsInfo(1);
      | for ii=1:numIn
      |     port_label('input',ii,'+')
      | end
  AddrAdjustConstant : Constant  Value=7  OutDataTypeStr=fixdt(0,4,0,'DataTypeOverride', 'Off')
  Compare To Constant : simulink/Logic and Bit Operations/Compare To Constant  relop===  const=fifo_size-1  OutDataTypeStr=boolean
  IncrConstant : Constant  OutDataTypeStr=fixdt(0,4,0,'DataTypeOverride', 'Off')
  Switch1 : Switch  Criteria=u2 ~= 0
  adjust_idx_mux : Switch  Criteria=u2 ~= 0
  dir_reg : Delay  DelayLength=1  InitialCondition=1
  idx_reg : Delay  DelayLength=1  InitialCondition=0
  idx : Outport
  wires:
  IncrConstant/1 -> adjust_idx_mux/3
  adjust_idx_mux/1 -> dir_reg/1
  dir_reg/1 -> AddSatOff/1(In1)
  action/1 -> Switch1/2  "actionProbe"
  idx_reg/1 -> idx/1, Switch1/3, AddSatOff/2(In2)  "origIdxidx"
  AddSatOff/1(Out) -> Switch1/1  "adjustedIdx"
  Switch1/1 -> Compare To Constant/1, idx_reg/1
  Compare To Constant/1 -> adjust_idx_mux/2
  AddrAdjustConstant/1 -> adjust_idx_mux/1

== system hdlsllibUNLOCKED/HDL RAMs/HDL FIFO/PushIdx ==
  action : Inport
  AddSatOff : Subsystem  mask(Add){OutDataTypeStr=fixdt(0,4,0,'DataTypeOverride', 'Off')}
      mask prompts: OutDataTypeStr "Output data type :"
      mask help: Add inputs. Overflows wrap to the minimum value that is representableby the data type.
      mask init:
      | hdlblkmask_fifo('addwrapoverflow');
      mask Display:
      | portsInfo = get_param(gcb, 'ports');
      | numIn = portsInfo(1);
      | for ii=1:numIn
      |     port_label('input',ii,'+')
      | end
  AddrAdjustConstant : Constant  Value=7  OutDataTypeStr=fixdt(0,4,0,'DataTypeOverride', 'Off')
  Compare To Constant : simulink/Logic and Bit Operations/Compare To Constant  relop===  const=fifo_size-1  OutDataTypeStr=boolean
  IncrConstant : Constant  OutDataTypeStr=fixdt(0,4,0,'DataTypeOverride', 'Off')
  Switch1 : Switch  Criteria=u2 ~= 0
  adjust_idx_mux : Switch  Criteria=u2 ~= 0
  dir_reg : Delay  DelayLength=1  InitialCondition=1
  idx_reg : Delay  DelayLength=1  InitialCondition=0
  idx : Outport
  wires:
  AddrAdjustConstant/1 -> adjust_idx_mux/1
  Compare To Constant/1 -> adjust_idx_mux/2
  Switch1/1 -> idx_reg/1, Compare To Constant/1
  AddSatOff/1(Out) -> Switch1/1  "adjustedIdx"
  idx_reg/1 -> idx/1, Switch1/3, AddSatOff/2(In2)  "origIdxidx"
  action/1 -> Switch1/2  "actionProbe"
  dir_reg/1 -> AddSatOff/1(In1)
  adjust_idx_mux/1 -> dir_reg/1
  IncrConstant/1 -> adjust_idx_mux/3

== system hdlsllibUNLOCKED/HDL RAMs/HDL FIFO/Upsample ==
  In : Inport
  Compare To Constant : simulink/Logic and Bit Operations/Compare To Constant  relop===  const=0  OutDataTypeStr=boolean
  Counter : simulink/Sources/Counter Limited  uplimit=(1/1) - 1  tsamp=-1
  Data Type Conversion Inherited : simulink/Signal Attributes/Data Type Conversion Inherited  ConvertRealWorld=Real World Value  DoSatur=off
      settings: SourceProductName=Simulink  SourceProductBaseCode=SL
  Gain : Gain  Gain=0  OutDataTypeStr=Inherit: Same as input
  Rate Transition : RateTransition  Integrity=off  OutPortSampleTimeOpt=Multiple of input port sample time  OutPortSampleTime=upVal
  Switch : Switch  Criteria=u2 ~= 0
  Terminator : Terminator
  Out : Outport
  wires:
  In/1 -> Rate Transition/1
  Rate Transition/1 -> Data Type Conversion Inherited/1, Switch/1, Gain/1
  Compare To Constant/1 -> Switch/2
  Switch/1 -> Out/1
  Gain/1 -> Switch/3
  Counter/1 -> Data Type Conversion Inherited/2, Compare To Constant/1
  Data Type Conversion Inherited/1 -> Terminator/1

== system hdlsllibUNLOCKED/HDL RAMs/HDL FIFO/Upsample1 ==
  In : Inport
  Compare To Constant : simulink/Logic and Bit Operations/Compare To Constant  relop===  const=0  OutDataTypeStr=boolean
  Counter : simulink/Sources/Counter Limited  uplimit=(1/1) - 1  tsamp=-1
  Data Type Conversion Inherited : simulink/Signal Attributes/Data Type Conversion Inherited  ConvertRealWorld=Real World Value  DoSatur=off
      settings: SourceProductName=Simulink  SourceProductBaseCode=SL
  Gain : Gain  Gain=0  OutDataTypeStr=Inherit: Same as input
  Rate Transition : RateTransition  Integrity=off  OutPortSampleTimeOpt=Multiple of input port sample time  OutPortSampleTime=upVal
  Switch : Switch  Criteria=u2 ~= 0
  Terminator : Terminator
  Out : Outport
  wires:
  Data Type Conversion Inherited/1 -> Terminator/1
  Counter/1 -> Compare To Constant/1, Data Type Conversion Inherited/2
  Gain/1 -> Switch/3
  Switch/1 -> Out/1
  Compare To Constant/1 -> Switch/2
  Rate Transition/1 -> Gain/1, Switch/1, Data Type Conversion Inherited/1
  In/1 -> Rate Transition/1

== system hdlsllibUNLOCKED/HDL RAMs/HDL FIFO/Upsample2 ==
  In : Inport
  Compare To Constant : simulink/Logic and Bit Operations/Compare To Constant  relop===  const=0  OutDataTypeStr=boolean
  Counter : simulink/Sources/Counter Limited  uplimit=ratio - 1  tsamp=-1
  Data Type Conversion Inherited : simulink/Signal Attributes/Data Type Conversion Inherited  ConvertRealWorld=Real World Value  DoSatur=off
      settings: SourceProductName=Simulink  SourceProductBaseCode=SL
  Gain : Gain  Gain=0  OutDataTypeStr=Inherit: Same as input
  Rate Transition : RateTransition  Integrity=off  OutPortSampleTimeOpt=Multiple of input port sample time  OutPortSampleTimeMultiple=1/ratio  OutPortSampleTime=upVal
  Switch : Switch  Criteria=u2 ~= 0
  Terminator : Terminator
  Out : Outport
  wires:
  In/1 -> Rate Transition/1
  Rate Transition/1 -> Data Type Conversion Inherited/1, Switch/1, Gain/1
  Compare To Constant/1 -> Switch/2
  Switch/1 -> Out/1
  Gain/1 -> Switch/3
  Counter/1 -> Data Type Conversion Inherited/2, Compare To Constant/1
  Data Type Conversion Inherited/1 -> Terminator/1

== system hdlsllibUNLOCKED/Sources/HDL Counter/Add_wrap ==
  step : Inport
  fb : Inport  Port=2
  Add : Sum  AccumDataTypeStr=fixdt(issigned,CountWordLen+1,0)  OutDataTypeStr=Inherit: Same as accumulator
  Mod_value : Constant  Value=2^CountWordLen  OutDataTypeStr=fixdt(0,CountWordLen+1,0,'DataTypeOverride','Off')
  Switch_wrap : Switch  Criteria=u2 > Threshold  Threshold=2^(CountWordLen-issigned)-1  OutDataTypeStr=fixdt(issigned,CountWordLen,0,'DataTypeOverride','Off')
  Wrap : Sum  Inputs=-+  AccumDataTypeStr=fixdt(1,CountWordLen+3,0)  OutDataTypeStr=Inherit: Same as accumulator
  add : Outport
  wires:
  Mod_value/1 -> Wrap/1
  Add/1 -> Switch_wrap/3, Switch_wrap/2, Wrap/2
  Wrap/1 -> Switch_wrap/1
  fb/1 -> Add/2
  Switch_wrap/1 -> add/1
  step/1 -> Add/1

== system hdlsllibUNLOCKED/Sources/HDL Counter/Dir_logic ==
  dir_port : Inport  OutDataTypeStr=boolean
  Logical Operator : Logic  Operator=XOR  AllPortsSameDT=off  OutDataTypeStr=boolean
  Pos_step : Constant  Value=(sign(CountStep) == 1)  OutDataTypeStr=boolean
  dn : Outport
  wires:
  dir_port/1 -> Logical Operator/1
  Pos_step/1 -> Logical Operator/2
  Logical Operator/1 -> dn/1

== system hdlsllibUNLOCKED/Sources/HDL Counter/Sub_wrap ==
  step : Inport
  fb : Inport  Port=2
  Add : Sum  Inputs=-+  AccumDataTypeStr=fixdt(1,CountWordLen+1,0)  OutDataTypeStr=Inherit: Same as accumulator
  Mod_value : Constant  Value=2^CountWordLen  OutDataTypeStr=fixdt(0,CountWordLen+1,0,'DataTypeOverride','Off')
  Switch_wrap : Switch  Threshold=-issigned*(2^(CountWordLen-1))  OutDataTypeStr=fixdt(issigned,CountWordLen,0,'DataTypeOverride','Off')
  Wrap : Sum  AccumDataTypeStr=fixdt(1,CountWordLen+3,0)  OutDataTypeStr=Inherit: Same as accumulator
  sub : Outport
  wires:
  Wrap/1 -> Switch_wrap/3
  Mod_value/1 -> Wrap/2
  Add/1 -> Switch_wrap/2, Switch_wrap/1, Wrap/1
  step/1 -> Add/1
  Switch_wrap/1 -> sub/1
  fb/1 -> Add/2

== system hdlsllibUNLOCKED/HDL Operations/Multiply-Accumulate/vectorMAC/Add ==
  note: 1) Add Subsystem or Model blocks as valid variant choices.
      | 2) You cannot connect blocks at this level. At simulation, connectivity is automatically
      | determined, based on the active variant and port name matching.
  In1 : Inport
  In2 : Inport  Port=2
  Add : Subsystem  VariantControl=nonzeroInitVal
  No Add : Subsystem  VariantControl=zeroInitVal
  Out1 : Outport

== system hdlsllibUNLOCKED/HDL RAMs/HDL FIFO/AdjustSampleOutNum/AddSatOff ==
  In1 : Inport
  In2 : Inport  Port=2
  Add : Sum  OutDataTypeStr=fixdt(0, 5, 0,'DataTypeOverride', 'Off')
  Bitwise Operator : simulink/Logic and Bit Operations/Bitwise Operator  logicop=AND  UseBitMask=on  BitMask=15  BitMaskRealWorld=Stored Integer
  Data Type Conversion : DataTypeConversion  OutDataTypeStr=fixdt(0,4,0,'DataTypeOverride', 'Off')
  Out : Outport
  wires:
  Data Type Conversion/1 -> Out/1
  Bitwise Operator/1 -> Data Type Conversion/1
  In1/1 -> Add/1
  In2/1 -> Add/2
  Add/1 -> Bitwise Operator/1

== system hdlsllibUNLOCKED/HDL RAMs/HDL FIFO/NextSampleOutNum/AddSatOff ==
  In1 : Inport
  In2 : Inport  Port=2
  Add : Sum  OutDataTypeStr=fixdt(0, 5, 0,'DataTypeOverride', 'Off')
  Bitwise Operator : simulink/Logic and Bit Operations/Bitwise Operator  logicop=AND  UseBitMask=on  BitMask=15  BitMaskRealWorld=Stored Integer
  Data Type Conversion : DataTypeConversion  OutDataTypeStr=fixdt(0,4,0,'DataTypeOverride', 'Off')
  Out : Outport
  wires:
  Data Type Conversion/1 -> Out/1
  Bitwise Operator/1 -> Data Type Conversion/1
  In1/1 -> Add/1
  In2/1 -> Add/2
  Add/1 -> Bitwise Operator/1

== system hdlsllibUNLOCKED/HDL RAMs/HDL FIFO/PopIdx/AddSatOff ==
  In1 : Inport
  In2 : Inport  Port=2
  Add : Sum  OutDataTypeStr=fixdt(0, 5, 0,'DataTypeOverride', 'Off')
  Bitwise Operator : simulink/Logic and Bit Operations/Bitwise Operator  logicop=AND  UseBitMask=on  BitMask=15  BitMaskRealWorld=Stored Integer
  Data Type Conversion : DataTypeConversion  OutDataTypeStr=fixdt(0,4,0,'DataTypeOverride', 'Off')
  Out : Outport
  wires:
  Data Type Conversion/1 -> Out/1
  Bitwise Operator/1 -> Data Type Conversion/1
  In1/1 -> Add/1
  In2/1 -> Add/2
  Add/1 -> Bitwise Operator/1

== system hdlsllibUNLOCKED/HDL RAMs/HDL FIFO/PushIdx/AddSatOff ==
  In1 : Inport
  In2 : Inport  Port=2
  Add : Sum  OutDataTypeStr=fixdt(0, 5, 0,'DataTypeOverride', 'Off')
  Bitwise Operator : simulink/Logic and Bit Operations/Bitwise Operator  logicop=AND  UseBitMask=on  BitMask=15  BitMaskRealWorld=Stored Integer
  Data Type Conversion : DataTypeConversion  OutDataTypeStr=fixdt(0,4,0,'DataTypeOverride', 'Off')
  Out : Outport
  wires:
  Data Type Conversion/1 -> Out/1
  Bitwise Operator/1 -> Data Type Conversion/1
  In1/1 -> Add/1
  In2/1 -> Add/2
  Add/1 -> Bitwise Operator/1

== system hdlsllibUNLOCKED/HDL Operations/Multiply-Accumulate/vectorMAC/Add/Add ==
  In1 : Inport
  In2 : Inport  Port=2
  Add : Sum  OutDataTypeStr=Inherit: Same as first input
  Out1 : Outport
  wires:
  In1/1 -> Add/1
  In2/1 -> Add/2
  Add/1 -> Out1/1

== system hdlsllibUNLOCKED/HDL Operations/Multiply-Accumulate/vectorMAC/Add/No Add ==
  In1 : Inport
  In2 : Inport  Port=2
  Terminator : Terminator
  Out1 : Outport
  wires:
  In1/1 -> Out1/1
  In2/1 -> Terminator/1

== matlab function hdlsllibUNLOCKED/HDL Operations/Serializer1D/EnumToIntConverter ==
  data: dataIn input; serializer_preProcessed output
function serializer_preProcessed = fcn(dataIn)
%#codegen
% added to support enum dataIn

if(coder.isenum(dataIn))  %is enum dataIn
    serializer_preProcessed = int32(dataIn);  %convert to int32
else
    serializer_preProcessed = dataIn;
end

== matlab function hdlsllibUNLOCKED/User-Defined Functions/MATLAB Function ==
  data: u input; y output
function y = fcn(u)
%#codegen

y = u;

== matlab function hdlsllibUNLOCKED/HDL Operations/Serializer1D/IntToEnumConverter ==
  data: dataIn input; serializer_PostProcessed output; dataOut input
function serializer_PostProcessed = fcn(dataIn, dataOut)
%#codegen
% added to support enum dataIn
if(coder.isenum(dataIn))  %is enum dataIn, convert dataOut back to enum
    EnumClassIn = class(dataIn);
    fh = str2func(EnumClassIn);
    serializer_PostProcessed = fh(dataOut);
else
    serializer_PostProcessed = dataOut;
end
